simulink model "dr_screening_pipeline"  (R2026a)
settings: Solver=VariableStepAuto  StopTime=28800
undefined symbols (not defined in the file or in its folder): DiscIntNeverNeededParam
libraries: simulink x2
settings Model: Creator=Abhij  LastModifiedBy=Abhij

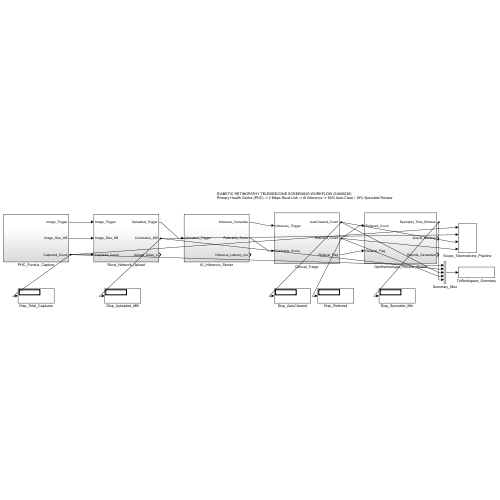
[thumbnail: Simulink's stored preview of the top-level diagram]
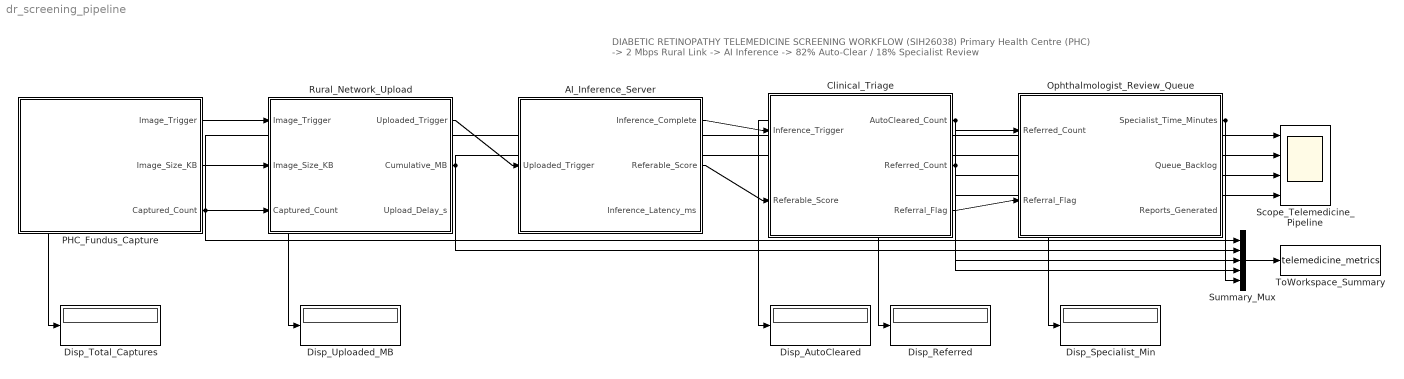
== system dr_screening_pipeline ==
  note: DIABETIC RETINOPATHY TELEMEDICINE SCREENING WORKFLOW (SIH26038)
      | Primary Health Centre (PHC) -> 2 Mbps Rural Link -> AI Inference -> 82% Auto-Clear / 18% Specialist Review
  AI_Inference_Server : Subsystem
  Clinical_Triage : Subsystem
  Disp_AutoCleared : Display
  Disp_Referred : Display
  Disp_Specialist_Min : Display
  Disp_Total_Captures : Display
  Disp_Uploaded_MB : Display
  Ophthalmologist_Review_Queue : Subsystem
  PHC_Fundus_Capture : Subsystem
  Rural_Network_Upload : Subsystem
  Scope_Telemedicine_Pipeline : Scope  NumInputPorts=4
  Summary_Mux : Mux  Inputs=5
  ToWorkspace_Summary : ToWorkspace  VariableName=telemedicine_metrics  SampleTime=-1
  wires:
  PHC_Fundus_Capture/1(Image_Trigger) -> Rural_Network_Upload/1(Image_Trigger)
  PHC_Fundus_Capture/2(Image_Size_KB) -> Rural_Network_Upload/2(Image_Size_KB)
  PHC_Fundus_Capture/3(Captured_Count) -> Rural_Network_Upload/3(Captured_Count), Disp_Total_Captures/1, Scope_Telemedicine_Pipeline/1, Summary_Mux/1
  Rural_Network_Upload/1(Uploaded_Trigger) -> AI_Inference_Server/1(Uploaded_Trigger)
  AI_Inference_Server/1(Inference_Complete) -> Clinical_Triage/1(Inference_Trigger)
  AI_Inference_Server/2(Referable_Score) -> Clinical_Triage/2(Referable_Score)
  Clinical_Triage/2(Referred_Count) -> Ophthalmologist_Review_Queue/1(Referred_Count), Disp_Referred/1, Scope_Telemedicine_Pipeline/4, Summary_Mux/4
  Clinical_Triage/3(Referral_Flag) -> Ophthalmologist_Review_Queue/2(Referral_Flag)
  Rural_Network_Upload/2(Cumulative_MB) -> Disp_Uploaded_MB/1, Scope_Telemedicine_Pipeline/2, Summary_Mux/2
  Clinical_Triage/1(AutoCleared_Count) -> Disp_AutoCleared/1, Scope_Telemedicine_Pipeline/3, Summary_Mux/3
  Ophthalmologist_Review_Queue/1(Specialist_Time_Minutes) -> Disp_Specialist_Min/1, Summary_Mux/5
  Summary_Mux/1 -> ToWorkspace_Summary/1

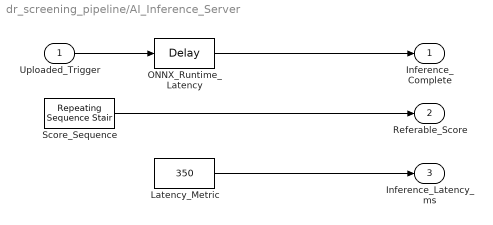
== system dr_screening_pipeline/AI_Inference_Server ==
  Uploaded_Trigger : Inport
  Latency_Metric : Constant  Value=350
  ONNX_Runtime_Latency : TransportDelay  DelayTime=0.35
  Score_Sequence : simulink/Sources/Repeating Sequence Stair  OutValues=[0.021 0.045 0.012 0.38 0.065 0.088 0.034 0.095 0.54 0.018 0.072 0.041 0.11 0.029 0.72 0.055 0.038 0.082 0.015 0.067 0.61 0.049 0.023 0.091 0.033 0.45 0.076 0.019 0.084 0.052 0.78 0.028 0.063 0.037 0.105 0.044 0.81 0.022 0.059 0.071 0.031 0.69 0.017 0.083 0.048 0.092 0.026 0.35 0.061 0.039]  tsamp=576  OutMin=[]  OutMax=[]  OutDataTypeStr=double  OutputDataTypeScalingMode=double  OutDataType=fixdt(0,8)  ConRadixGroup=Best Precision: Vector-wise  OutScaling=2^-12
  Inference_Complete : Outport
  Referable_Score : Outport  Port=2
  Inference_Latency_ms : Outport  Port=3
  wires:
  Uploaded_Trigger/1 -> ONNX_Runtime_Latency/1
  ONNX_Runtime_Latency/1 -> Inference_Complete/1
  Score_Sequence/1 -> Referable_Score/1
  Latency_Metric/1 -> Inference_Latency_ms/1

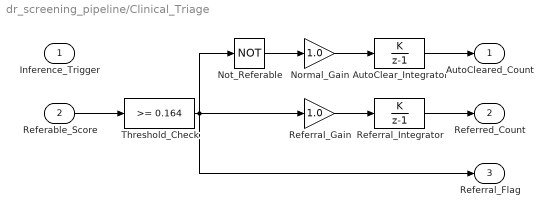
== system dr_screening_pipeline/Clinical_Triage ==
  Inference_Trigger : Inport
  Referable_Score : Inport  Port=2
  AutoClear_Integrator : DiscreteIntegrator  IntegratorMethod=Accumulation: Forward Euler  SampleTime=576  OutDataTypeStr=double  ICPrevOutput=DiscIntNeverNeededParam  ICPrevScaledInput=DiscIntNeverNeededParam
  Normal_Gain : Gain  Gain=1.0
  Not_Referable : Logic  Operator=NOT  AllPortsSameDT=off  OutDataTypeStr=boolean
  Referral_Gain : Gain  Gain=1.0
  Referral_Integrator : DiscreteIntegrator  IntegratorMethod=Accumulation: Forward Euler  SampleTime=576  OutDataTypeStr=double  ICPrevOutput=DiscIntNeverNeededParam  ICPrevScaledInput=DiscIntNeverNeededParam
  Threshold_Check : simulink/Logic and Bit Operations/Compare To Constant  relop=>=  const=0.164  OutDataTypeStr=boolean
  AutoCleared_Count : Outport
  Referred_Count : Outport  Port=2
  Referral_Flag : Outport  Port=3
  wires:
  Referable_Score/1 -> Threshold_Check/1
  Threshold_Check/1 -> Not_Referable/1, Referral_Gain/1, Referral_Flag/1
  Not_Referable/1 -> Normal_Gain/1
  Normal_Gain/1 -> AutoClear_Integrator/1
  AutoClear_Integrator/1 -> AutoCleared_Count/1
  Referral_Gain/1 -> Referral_Integrator/1
  Referral_Integrator/1 -> Referred_Count/1

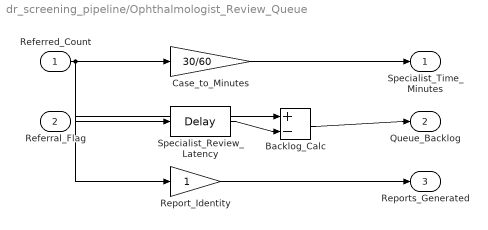
== system dr_screening_pipeline/Ophthalmologist_Review_Queue ==
  Referred_Count : Inport
  Referral_Flag : Inport  Port=2
  Backlog_Calc : Sum  Inputs=+-
  Case_to_Minutes : Gain  Gain=30/60
  Report_Identity : Gain
  Specialist_Review_Latency : TransportDelay  DelayTime=30.0
  Specialist_Time_Minutes : Outport
  Queue_Backlog : Outport  Port=2
  Reports_Generated : Outport  Port=3
  wires:
  Referred_Count/1 -> Case_to_Minutes/1, Backlog_Calc/1, Specialist_Review_Latency/1, Report_Identity/1
  Case_to_Minutes/1 -> Specialist_Time_Minutes/1
  Specialist_Review_Latency/1 -> Backlog_Calc/2
  Backlog_Calc/1 -> Queue_Backlog/1
  Report_Identity/1 -> Reports_Generated/1

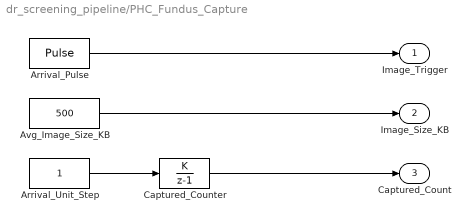
== system dr_screening_pipeline/PHC_Fundus_Capture ==
  Arrival_Pulse : DiscretePulseGenerator  PulseType=Time based  Period=576
  Arrival_Unit_Step : Constant  SampleTime=576
  Avg_Image_Size_KB : Constant  Value=500
  Captured_Counter : DiscreteIntegrator  IntegratorMethod=Accumulation: Forward Euler  SampleTime=576  OutDataTypeStr=double  ICPrevOutput=DiscIntNeverNeededParam  ICPrevScaledInput=DiscIntNeverNeededParam
  Image_Trigger : Outport
  Image_Size_KB : Outport  Port=2
  Captured_Count : Outport  Port=3
  wires:
  Arrival_Pulse/1 -> Image_Trigger/1
  Avg_Image_Size_KB/1 -> Image_Size_KB/1
  Arrival_Unit_Step/1 -> Captured_Counter/1
  Captured_Counter/1 -> Captured_Count/1

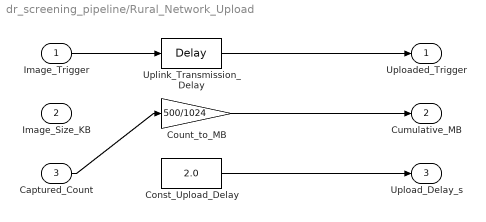
== system dr_screening_pipeline/Rural_Network_Upload ==
  Image_Trigger : Inport
  Image_Size_KB : Inport  Port=2
  Captured_Count : Inport  Port=3
  Const_Upload_Delay : Constant  Value=2.0
  Count_to_MB : Gain  Gain=500/1024
  Uplink_Transmission_Delay : TransportDelay  DelayTime=2.0
  Uploaded_Trigger : Outport
  Cumulative_MB : Outport  Port=2
  Upload_Delay_s : Outport  Port=3
  wires:
  Image_Trigger/1 -> Uplink_Transmission_Delay/1
  Uplink_Transmission_Delay/1 -> Uploaded_Trigger/1
  Captured_Count/1 -> Count_to_MB/1
  Count_to_MB/1 -> Cumulative_MB/1
  Const_Upload_Delay/1 -> Upload_Delay_s/1
